simulink model "pidcontroller"  (R2023b)
settings: Solver=VariableStepAuto  StartTime=0.0  StopTime=30.0  RelTol=1e-3
settings Model: Creator=25446  LastModifiedBy=25446

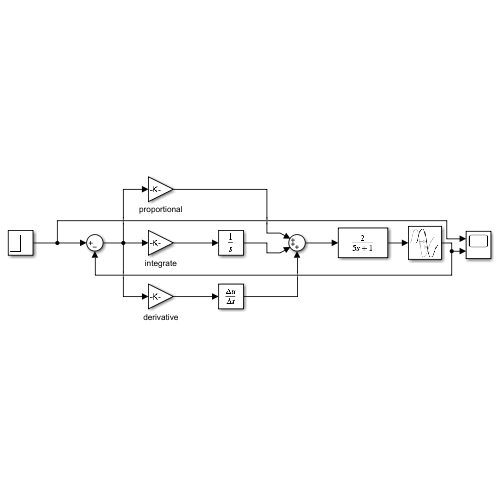
[thumbnail: Simulink's stored preview of the top-level diagram]
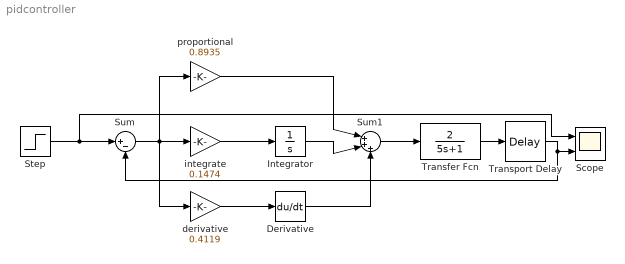
== system pidcontroller ==
  Derivative : Derivative
  Integrator : Integrator
  Scope : Scope  NumInputPorts=2
  Step : Step  SampleTime=0
  Sum : Sum  Inputs=|+-
  Sum1 : Sum  Inputs=|+++
  Transfer Fcn : TransferFcn  Numerator=[2]  Denominator=[5 1]
  Transport Delay : TransportDelay  DelayTime=2
  derivative : Gain  Gain=0.4119
  integrate : Gain  Gain=0.1474
  proportional : Gain  Gain=0.8935
  wires:
  Sum/1 -> derivative/1, proportional/1, integrate/1
  integrate/1 -> Integrator/1
  derivative/1 -> Derivative/1
  Step/1 -> Scope/1, Sum/1
  proportional/1 -> Sum1/1
  Integrator/1 -> Sum1/2
  Derivative/1 -> Sum1/3
  Sum1/1 -> Transfer Fcn/1
  Transport Delay/1 -> Sum/2, Scope/2
  Transfer Fcn/1 -> Transport Delay/1
